simulink model "sedemo_absbrake_can"  (Simulink 7.5)
settings: Solver=ode45  SolverMode=SingleTasking  StartTime=0.0  StopTime=17  MaxStep=inf  RelTol=2e-2  AbsTol=1e-4
PreLoadFcn:
  | sedemo_absdata;
  | BUSCapacity = 50000;
StopFcn:
  | if exist ('logsout')
  | tagName = 'Net';
  | sedemo_absbrakeplots_delay;
  | clear figExt tagName;
  | end
values from neighbouring files (symbols this model uses):
  ctrl = 1    [sedemo_absdata.m]
  g = 32.18    [sedemo_absdata.m]
  I = 5    [sedemo_absdata.m]
  Kf = 1    [sedemo_absdata.m]
  m = 50    [sedemo_absdata.m]
  mu = [0 .4 .8 .97 1.0 .98 .96 .94 .92 .9 .88 .855 .83 .81 .79 .77 .75 .73 .72 .71 .7]    [sedemo_absdata.m]
  PBmax = 1500    [sedemo_absdata.m]
  Rr = 15/12    (= 1.25)    [sedemo_absdata.m]
  slip = (0:.05:1.0)    [sedemo_absdata.m]
  TB = 0.01    [sedemo_absdata.m]
  v0 = 88    [sedemo_absdata.m]
undefined symbols (not defined in the file or in its folder): des_subsystemblock, des_subsysteminport, des_subsystemoutport, des_subsystemsupportblock
libraries: simeventsrouting1 x30, simeventstranslate1 x25, simeventssink1 x21, simeventsserver1 x19, simeventsattributes2 x15, simeventsgates1 x10, simeventsqueue1 x6, simulink x5, simeventsgenerators1 x5, simeventssignalmanage1 x5, simeventstiming1 x3, simeventsinfo x1
(part 2 of 4)

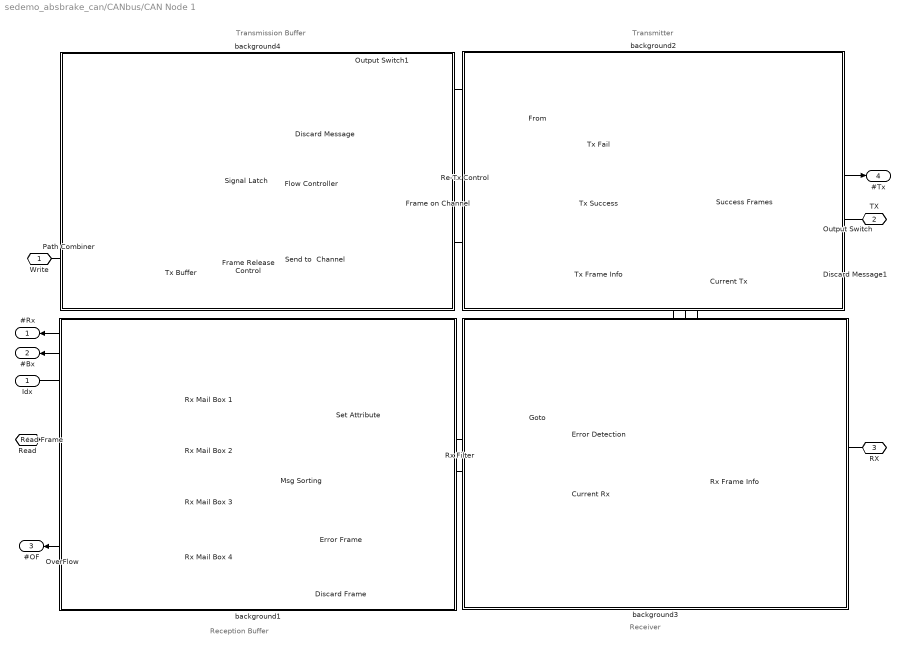
== system sedemo_absbrake_can/CANbus/CAN Node 1 ==
  note: Receiver
  note: Transmitter
  note: Transmission Buffer
  note: Reception Buffer
  Idx : Inport  OutDataType=sfix(16)  OutScaling=2^0
  Current Rx : simeventsserver1/Single Server  Priority=1  SystemSampleTime=-1  ServiceTimeFrom=Dialog  ServiceTime=0  AttributeName=ServiceTime  PriorityServiceCompletion=2400  PermitPreemption=off  SortingAttributeName=ID  SortingDirection=Ascending  WriteToAttribute=off  ResidualAttributeName=ResidualServiceTime  CreateAttribute=on  EnableTOPort=off  StatNumberDeparted=Off  StatNumberInBlock=Off  StatNumberPreempted=Off  StatPendingEntity=Off  StatAverageWait=Off  StatUtilization=Off  StatNumberTimedout=Off
  Current Tx : simeventsserver1/Single Server  Priority=1  SystemSampleTime=-1  ServiceTimeFrom=Dialog  ServiceTime=0  AttributeName=ServiceTime  PriorityServiceCompletion=2400  PermitPreemption=off  SortingAttributeName=ID  SortingDirection=Ascending  WriteToAttribute=off  ResidualAttributeName=ResidualServiceTime  CreateAttribute=on  EnableTOPort=off  StatNumberDeparted=Off  StatNumberInBlock=Off  StatNumberPreempted=Off  StatPendingEntity=Off  StatAverageWait=Off  StatUtilization=Off  StatNumberTimedout=Off
  Discard Message1 : simeventssink1/Entity Sink  Priority=1  SystemSampleTime=-1  AvailableForArrivals=on  StatNumberArrived=Off
  Discard Frame : simeventssink1/Entity Sink  Priority=1  SystemSampleTime=-1  AvailableForArrivals=on  StatNumberArrived=Off
  Discard Message : simeventssink1/Entity Sink  Priority=1  SystemSampleTime=-1  AvailableForArrivals=on  StatNumberArrived=Off
  Error Detection : Subsystem  LoadFcn=des_subsystemblock(gcb, 'load');  InitFcn=des_subsystemblock(gcb, 'init');  StartFcn=des_subsystemblock(gcb, 'start');  StopFcn=des_subsystemblock(gcb, 'stop');
      settings: CopyFcn=des_subsystemblock(gcb, 'copy');  DeleteFcn=des_subsystemblock(gcb, 'delete');  UndoDeleteFcn=des_subsystemblock(gcb, 'undodelete');  ModelCloseFcn=des_subsystemblock(gcb, 'modelclose');  PreSaveFcn=des_subsystemblock(gcb, 'presave');  NameChangeFcn=des_subsystemblock(gcb, 'namechange');  ParentCloseFcn=des_subsystemblock(gcb, 'parentclose');  ErrorFcn=des_subsystemerror
  Error Frame : simeventssink1/Entity Sink  Priority=1  SystemSampleTime=-1  AvailableForArrivals=on  StatNumberArrived=Off
  Flow Controller : Subsystem  LoadFcn=des_subsystemblock(gcb, 'load');  InitFcn=des_subsystemblock(gcb, 'init');  StartFcn=des_subsystemblock(gcb, 'start');  StopFcn=des_subsystemblock(gcb, 'stop');
      settings: CopyFcn=des_subsystemblock(gcb, 'copy');  DeleteFcn=des_subsystemblock(gcb, 'delete');  UndoDeleteFcn=des_subsystemblock(gcb, 'undodelete');  ModelCloseFcn=des_subsystemblock(gcb, 'modelclose');  PreSaveFcn=des_subsystemblock(gcb, 'presave');  NameChangeFcn=des_subsystemblock(gcb, 'namechange');  ParentCloseFcn=des_subsystemblock(gcb, 'parentclose');  ErrorFcn=des_subsystemerror
  Frame Release Control : simeventsgates1/Enabled Gate  Priority=1  SystemSampleTime=-1  SpecifyEventPriority=on  PriorityGateEnableOpenClose=2300  StatNumberDeparted=Off
  Frame on Channel : simeventsqueue1/FIFO Queue  Priority=1  SystemSampleTime=-1  Capacity=2  EnableTOPort=off  StatNumberDeparted=Off  StatNumberInBlock=On  StatPendingEntity=Off  StatAverageWait=Off  StatAverageQueueLength=Off  StatNumberTimedout=Off
  Msg Sorting : simeventsrouting1/Output Switch  Priority=1  SystemSampleTime=-1  NumberOutputPorts=4  SwitchingCriterion=Round robin  InitialSeed=34567  AttributeName=Attribute1  InitialConditionsOpt=off  InitialConditions=1  EntityBufferOpt=off  SpecifyEventPriority=off  PriorityOutputSwitchSelectPort=4100  TimeoutPortOpt=off  StatNumberDeparted=On  StatNumberTimedOut=Off  StatPendingEntity=Off  StatLastDeparturePort=On  EvaluatedNumPorts=4
  Output Switch : simeventsrouting1/Output Switch  Priority=1  SystemSampleTime=-1  NumberOutputPorts=2  SwitchingCriterion=First port that is not blocked  InitialSeed=34567  AttributeName=Attribute1  InitialConditionsOpt=off  InitialConditions=1  EntityBufferOpt=off  SpecifyEventPriority=off  PriorityOutputSwitchSelectPort=4100  TimeoutPortOpt=off  StatNumberDeparted=Off  StatNumberTimedOut=Off  StatPendingEntity=Off  StatLastDeparturePort=Off  EvaluatedNumPorts=2
  Output Switch1 : simeventsrouting1/Output Switch  Priority=1  SystemSampleTime=-1  NumberOutputPorts=2  SwitchingCriterion=First port that is not blocked  InitialSeed=34567  AttributeName=Attribute1  InitialConditionsOpt=off  InitialConditions=1  EntityBufferOpt=off  SpecifyEventPriority=off  PriorityOutputSwitchSelectPort=4100  TimeoutPortOpt=off  StatNumberDeparted=Off  StatNumberTimedOut=Off  StatPendingEntity=Off  StatLastDeparturePort=Off  EvaluatedNumPorts=2
  OverFlow : simeventsrouting1/Path Combiner  Priority=1  SystemSampleTime=-1  NumberInputPorts=4  InputPortPrecedence=IN1 port  InitialSeed=45675  SpecifyEventPriority=off  PriorityPathCombinerPortPrecedenceSelection=4100  StatNumberDeparted=On  StatLastArrivalPort=Off  EvaluatedNumPorts=4
  Path Combiner : simeventsrouting1/Path Combiner  Priority=1  SystemSampleTime=-1  NumberInputPorts=2  InputPortPrecedence=IN1 port  InitialSeed=45675  SpecifyEventPriority=off  PriorityPathCombinerPortPrecedenceSelection=4100  StatNumberDeparted=Off  StatLastArrivalPort=Off  EvaluatedNumPorts=2
  Re-Tx Control : simeventsrouting1/Output Switch  Priority=1  SystemSampleTime=-1  NumberOutputPorts=2  SwitchingCriterion=First port that is not blocked  InitialSeed=34567  AttributeName=Attribute1  InitialConditionsOpt=off  InitialConditions=1  EntityBufferOpt=off  SpecifyEventPriority=off  PriorityOutputSwitchSelectPort=4100  TimeoutPortOpt=off  StatNumberDeparted=Off  StatNumberTimedOut=Off  StatPendingEntity=Off  StatLastDeparturePort=Off  EvaluatedNumPorts=2
  Read Frame : simeventsrouting1/Input Switch  Priority=1  SystemSampleTime=-1  NumberInputPorts=4  SwitchingCriterion=From signal port p  InitialSeed=23453  SpecifyEventPriority=off  PriorityInputSwitchSelectPort=4000  StatNumberDeparted=Off  StatLastArrivalPort=Off  EvaluatedNumPorts=4
  Rx Filter : simeventsrouting1/Output Switch  Priority=1  SystemSampleTime=-1  NumberOutputPorts=3  SwitchingCriterion=From signal port p  InitialSeed=34567  AttributeName=Attribute1  InitialConditionsOpt=off  InitialConditions=1  EntityBufferOpt=off  SpecifyEventPriority=off  PriorityOutputSwitchSelectPort=4100  TimeoutPortOpt=off  StatNumberDeparted=On  StatNumberTimedOut=Off  StatPendingEntity=Off  StatLastDeparturePort=Off  EvaluatedNumPorts=3
  Rx Frame Info : simeventsattributes2/Get Attribute  Priority=1  DialogController=des_ddg_create  DialogControllerArgs=DataTag128  SystemSampleTime=-1  AttributeName=ID|RndLoss|RTR|Data  AttributeMissing=Error|Error|Error|Error  AttributeDefaultValue=1|1|1|1  AttributeSendTiming=After entity departure|After entity departure|After entity departure|After entity departure  AttributeTreatAsVector=1|1|1|1  StatNumberDeparted=Off  EvaluatedDefaultAttributeValue={[];[];[];[]}
  Rx Mail Box {1..4} (4 alike) : simeventsserver1/Single Server  Priority=1  SystemSampleTime=-1  ServiceTimeFrom=Dialog  ServiceTime=0  AttributeName=ServiceTime  PriorityServiceCompletion=2400  PermitPreemption=on  SortingAttributeName=time  SortingDirection=Descending  WriteToAttribute=off  ResidualAttributeName=ResidualServiceTime  CreateAttribute=on  EnableTOPort=off  StatNumberDeparted=Off  StatNumberInBlock=Off  StatNumberPreempted=Off  StatPendingEntity=Off  StatAverageWait=Off  StatUtilization=Off  StatNumberTimedout=Off
  Send to  Channel : simeventsrouting1/Replicate  Priority=1  SystemSampleTime=-1  NumberOutputPorts=2  ReplicateEntityWhen=All entity output ports are not blocked  OutputPortPrecedence=OUT1 port  InitialSeed=56789  ActionUponBlocking=Discard entity  StatNumberArrived=Off  StatNumberDeparted=Off  EvaluatedNumPorts=2
  Set Attribute : simeventsattributes2/Set Attribute  Priority=1  DialogController=des_ddg_create  DialogControllerArgs=DataTag135  SystemSampleTime=-1  AttributeFrom=Signal port  AttributeName=time  AttributeTreatAsVector=1  AttributeValue=1  AttributeCreate=on  StatNumberDeparted=Off  EvaluatedAttributeValue={[]}
  Signal Latch : simeventssignalmanage1/Signal Latch  Priority=1  SystemSampleTime=-1  InitialMemoryValue=1  WriteMemoryUpon=Sample time hit from port wts  MemoryWriteEdgeOption=Either  SpecifyWriteEventPriority=on  PriorityMemoryWrite=2200  ReadMemoryUpon=Write to memory event  MemoryReadEdgeOption=Falling  SpecifyReadEventPriority=on  PriorityMemoryRead=7000  ReportMemoryState=off  ReportMemoryUponWrite=off  ReportMemoryUponRead=on
  Success Frames : simeventssink1/Entity Sink  Priority=1  SystemSampleTime=-1  AvailableForArrivals=on  StatNumberArrived=On
  Tx Buffer : simeventsqueue1/Priority Queue  Priority=1  SystemSampleTime=-1  Capacity=15  SortingAttributeName=ID  SortingDirection=Ascending  EnableTOPort=off  StatNumberDeparted=Off  StatNumberInBlock=Off  StatPendingEntity=Off  StatAverageWait=Off  StatAverageQueueLength=Off  StatNumberTimedout=Off
  Tx Fail : simeventsgates1/Release Gate  Priority=1  SystemSampleTime=-1  OpenGateUpon=Change in signal from port vc  SignalEdgeOption=Falling  SpecifyEventPriority=on  PriorityGateRelease=2000  StatNumberDeparted=Off
  Tx Frame Info : simeventsattributes2/Get Attribute  Priority=1  DialogController=des_ddg_create  DialogControllerArgs=DataTag141  SystemSampleTime=-1  AttributeName=ID|RTR|Data  AttributeMissing=Error|Error|Error  AttributeDefaultValue=1|1|1  AttributeSendTiming=After entity departure|After entity departure|After entity departure  AttributeTreatAsVector=1|1|1  StatNumberDeparted=Off  EvaluatedDefaultAttributeValue={[];[];[]}
  Tx Success : simeventsgates1/Release Gate  Priority=1  SystemSampleTime=-1  OpenGateUpon=Change in signal from port vc  SignalEdgeOption=Rising  SpecifyEventPriority=on  PriorityGateRelease=2000  StatNumberDeparted=Off
  background1 : Subsystem
      mask Display: disp('')
  background2 : Subsystem
      mask Display: disp('')
  background3 : Subsystem
      mask Display: disp('')
  background4 : Subsystem
      mask Display: disp('')
  Write : PMIOPort  Port=1  Side=Right
  TX : PMIOPort  Port=2  Side=Left
  RX : PMIOPort  Port=3  Side=Left
  Read : PMIOPort  Port=4  Side=Right
  #Rx : Outport  OutDataType=sfix(16)  OutScaling=2^0
  #Bx : Outport  Port=2  OutDataType=sfix(16)  OutScaling=2^0
  #OF : Outport  Port=3  OutDataType=sfix(16)  OutScaling=2^0
  #Tx : Outport  Port=4  OutDataType=sfix(16)  OutScaling=2^0
  wires:
  [Ack] -> Tx Success/1, Tx Fail/1
  Error Detection/2(ACK) -> [Ack]
  Error Detection/1(Idx) -> Rx Filter/1
  Rx Frame Info/4 -> Error Detection/4(Rx_Data)
  Rx Frame Info/3 -> Error Detection/3(Rx_RTR)
  Tx Frame Info/1 -> Error Detection/5(Tx_ID)
  Tx Frame Info/2 -> Error Detection/6(Tx_RTR)
  Tx Frame Info/3 -> Error Detection/7(Tx_Data)
  Rx Frame Info/2 -> Error Detection/2(Loss)
  Rx Frame Info/1 -> Error Detection/1(Rx_ID)
  Rx Filter/1 -> Set Attribute/1
  Frame on Channel/1 -> Flow Controller/1(busy)
  Idx/1 -> Read Frame/1
  Msg Sorting/2 -> #Bx/1
  OverFlow/1 -> #OF/1
  Msg Sorting/1 -> #Rx/1
  Success Frames/1 -> #Tx/1
  Flow Controller/1(en) -> Signal Latch/1, Signal Latch/2
  Signal Latch/1 -> Frame Release Control/1
  connections:
  Tx Frame Info/RConn1 -- Current Tx/LConn1
  Current Tx/RConn1 -- Output Switch/LConn1
  Send to  Channel/RConn1 -- Frame on Channel/LConn1
  Send to  Channel/RConn2 -- Tx Frame Info/LConn1
  RX/RConn1 -- Rx Frame Info/LConn1
  Rx Mail Box 4/RConn1 -- Read Frame/LConn4
  Rx Mail Box 3/RConn1 -- Read Frame/LConn3
  Rx Mail Box 2/RConn1 -- Read Frame/LConn2
  Rx Mail Box 1/RConn1 -- Read Frame/LConn1
  Rx Mail Box 1/RConn2 -- OverFlow/LConn1
  Rx Mail Box 2/RConn2 -- OverFlow/LConn2
  Rx Mail Box 3/RConn2 -- OverFlow/LConn3
  Rx Mail Box 4/RConn2 -- OverFlow/LConn4
  Rx Frame Info/RConn1 -- Current Rx/LConn1
  Output Switch1/RConn1 -- Path Combiner/LConn1
  Tx Fail/RConn1 -- Output Switch1/LConn1
  Output Switch/RConn1 -- TX/RConn1
  Set Attribute/RConn1 -- Msg Sorting/LConn1
  Rx Filter/RConn1 -- Set Attribute/LConn1
  Rx Filter/RConn3 -- Discard Frame/LConn1
  Tx Success/RConn1 -- Success Frames/LConn1
  Write/RConn1 -- Path Combiner/LConn2
  Path Combiner/RConn1 -- Tx Buffer/LConn1
  Frame Release Control/RConn1 -- Send to  Channel/LConn1
  Tx Buffer/RConn1 -- Frame Release Control/LConn1
  Re-Tx Control/RConn1 -- Tx Fail/LConn1
  Re-Tx Control/RConn2 -- Tx Success/LConn1
  Frame on Channel/RConn1 -- Re-Tx Control/LConn1
  Current Rx/RConn1 -- Rx Filter/LConn1
  Rx Filter/RConn2 -- Error Frame/LConn1
  Msg Sorting/RConn1 -- Rx Mail Box 1/LConn1
  Msg Sorting/RConn2 -- Rx Mail Box 2/LConn1
  Msg Sorting/RConn3 -- Rx Mail Box 3/LConn1
  Msg Sorting/RConn4 -- Rx Mail Box 4/LConn1
  Read Frame/RConn1 -- Read/RConn1
  Output Switch/RConn2 -- Discard Message1/LConn1
  Discard Message/LConn1 -- Output Switch1/RConn2

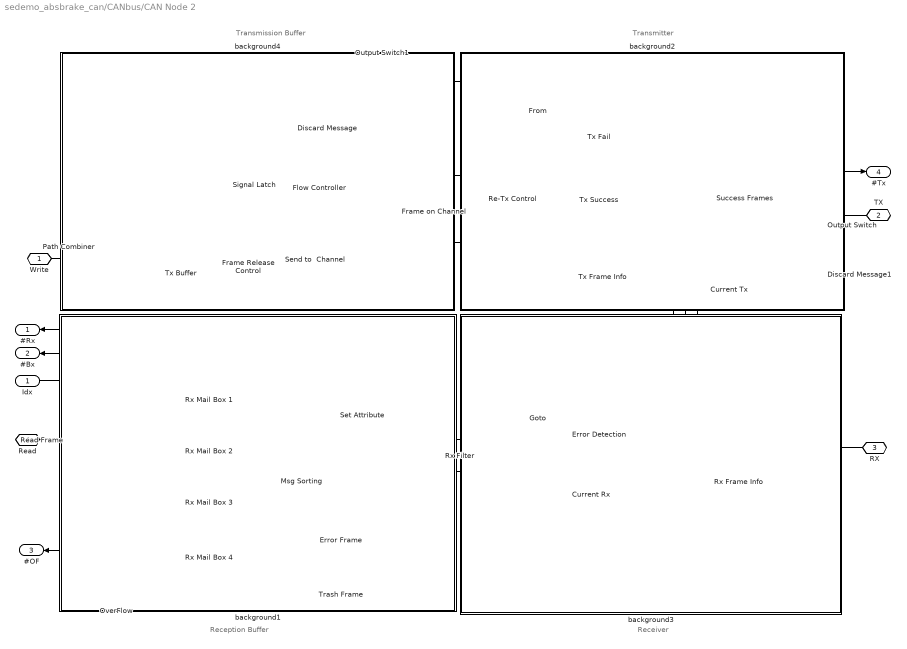
== system sedemo_absbrake_can/CANbus/CAN Node 2 ==
  note: Receiver
  note: Transmitter
  note: Transmission Buffer
  note: Reception Buffer
  Idx : Inport  OutDataType=sfix(16)  OutScaling=2^0
  Current Rx : simeventsserver1/Single Server  Priority=1  SystemSampleTime=-1  ServiceTimeFrom=Dialog  ServiceTime=0  AttributeName=ServiceTime  PriorityServiceCompletion=2400  PermitPreemption=off  SortingAttributeName=ID  SortingDirection=Ascending  WriteToAttribute=off  ResidualAttributeName=ResidualServiceTime  CreateAttribute=on  EnableTOPort=off  StatNumberDeparted=Off  StatNumberInBlock=Off  StatNumberPreempted=Off  StatPendingEntity=Off  StatAverageWait=Off  StatUtilization=Off  StatNumberTimedout=Off
  Current Tx : simeventsserver1/Single Server  Priority=1  SystemSampleTime=-1  ServiceTimeFrom=Dialog  ServiceTime=0  AttributeName=ServiceTime  PriorityServiceCompletion=2400  PermitPreemption=off  SortingAttributeName=ID  SortingDirection=Ascending  WriteToAttribute=off  ResidualAttributeName=ResidualServiceTime  CreateAttribute=on  EnableTOPort=off  StatNumberDeparted=Off  StatNumberInBlock=Off  StatNumberPreempted=Off  StatPendingEntity=Off  StatAverageWait=Off  StatUtilization=Off  StatNumberTimedout=Off
  Discard Message : simeventssink1/Entity Sink  Priority=1  SystemSampleTime=-1  AvailableForArrivals=on  StatNumberArrived=Off
  Discard Message1 : simeventssink1/Entity Sink  Priority=1  SystemSampleTime=-1  AvailableForArrivals=on  StatNumberArrived=Off
  Error Detection : Subsystem  LoadFcn=des_subsystemblock(gcb, 'load');  InitFcn=des_subsystemblock(gcb, 'init');  StartFcn=des_subsystemblock(gcb, 'start');  StopFcn=des_subsystemblock(gcb, 'stop');
      settings: CopyFcn=des_subsystemblock(gcb, 'copy');  DeleteFcn=des_subsystemblock(gcb, 'delete');  UndoDeleteFcn=des_subsystemblock(gcb, 'undodelete');  ModelCloseFcn=des_subsystemblock(gcb, 'modelclose');  PreSaveFcn=des_subsystemblock(gcb, 'presave');  NameChangeFcn=des_subsystemblock(gcb, 'namechange');  ParentCloseFcn=des_subsystemblock(gcb, 'parentclose');  ErrorFcn=des_subsystemerror
  Error Frame : simeventssink1/Entity Sink  Priority=1  SystemSampleTime=-1  AvailableForArrivals=on  StatNumberArrived=Off
  Flow Controller : Subsystem  LoadFcn=des_subsystemblock(gcb, 'load');  InitFcn=des_subsystemblock(gcb, 'init');  StartFcn=des_subsystemblock(gcb, 'start');  StopFcn=des_subsystemblock(gcb, 'stop');
      settings: CopyFcn=des_subsystemblock(gcb, 'copy');  DeleteFcn=des_subsystemblock(gcb, 'delete');  UndoDeleteFcn=des_subsystemblock(gcb, 'undodelete');  ModelCloseFcn=des_subsystemblock(gcb, 'modelclose');  PreSaveFcn=des_subsystemblock(gcb, 'presave');  NameChangeFcn=des_subsystemblock(gcb, 'namechange');  ParentCloseFcn=des_subsystemblock(gcb, 'parentclose');  ErrorFcn=des_subsystemerror
  Frame Release Control : simeventsgates1/Enabled Gate  Priority=1  SystemSampleTime=-1  SpecifyEventPriority=on  PriorityGateEnableOpenClose=2300  StatNumberDeparted=Off
  Frame on Channel : simeventsqueue1/FIFO Queue  Priority=1  SystemSampleTime=-1  Capacity=2  EnableTOPort=off  StatNumberDeparted=Off  StatNumberInBlock=On  StatPendingEntity=Off  StatAverageWait=Off  StatAverageQueueLength=Off  StatNumberTimedout=Off
  Msg Sorting : simeventsrouting1/Output Switch  Priority=1  SystemSampleTime=-1  NumberOutputPorts=4  SwitchingCriterion=Round robin  InitialSeed=34567  AttributeName=Attribute1  InitialConditionsOpt=off  InitialConditions=1  EntityBufferOpt=off  SpecifyEventPriority=off  PriorityOutputSwitchSelectPort=4100  TimeoutPortOpt=off  StatNumberDeparted=On  StatNumberTimedOut=Off  StatPendingEntity=Off  StatLastDeparturePort=On  EvaluatedNumPorts=4
  Output Switch : simeventsrouting1/Output Switch  Priority=1  SystemSampleTime=-1  NumberOutputPorts=2  SwitchingCriterion=First port that is not blocked  InitialSeed=34567  AttributeName=Attribute1  InitialConditionsOpt=off  InitialConditions=1  EntityBufferOpt=off  SpecifyEventPriority=off  PriorityOutputSwitchSelectPort=4100  TimeoutPortOpt=off  StatNumberDeparted=Off  StatNumberTimedOut=Off  StatPendingEntity=Off  StatLastDeparturePort=Off  EvaluatedNumPorts=2
  Output Switch1 : simeventsrouting1/Output Switch  Priority=1  SystemSampleTime=-1  NumberOutputPorts=2  SwitchingCriterion=First port that is not blocked  InitialSeed=34567  AttributeName=Attribute1  InitialConditionsOpt=off  InitialConditions=1  EntityBufferOpt=off  SpecifyEventPriority=off  PriorityOutputSwitchSelectPort=4100  TimeoutPortOpt=off  StatNumberDeparted=Off  StatNumberTimedOut=Off  StatPendingEntity=Off  StatLastDeparturePort=Off  EvaluatedNumPorts=2
  OverFlow : simeventsrouting1/Path Combiner  Priority=1  SystemSampleTime=-1  NumberInputPorts=4  InputPortPrecedence=IN1 port  InitialSeed=45675  SpecifyEventPriority=off  PriorityPathCombinerPortPrecedenceSelection=4100  StatNumberDeparted=On  StatLastArrivalPort=Off  EvaluatedNumPorts=4
  Path Combiner : simeventsrouting1/Path Combiner  Priority=1  SystemSampleTime=-1  NumberInputPorts=2  InputPortPrecedence=IN1 port  InitialSeed=45675  SpecifyEventPriority=off  PriorityPathCombinerPortPrecedenceSelection=4100  StatNumberDeparted=Off  StatLastArrivalPort=Off  EvaluatedNumPorts=2
  Re-Tx Control : simeventsrouting1/Output Switch  Priority=1  SystemSampleTime=-1  NumberOutputPorts=2  SwitchingCriterion=First port that is not blocked  InitialSeed=34567  AttributeName=Attribute1  InitialConditionsOpt=off  InitialConditions=1  EntityBufferOpt=off  SpecifyEventPriority=off  PriorityOutputSwitchSelectPort=4100  TimeoutPortOpt=off  StatNumberDeparted=Off  StatNumberTimedOut=Off  StatPendingEntity=Off  StatLastDeparturePort=Off  EvaluatedNumPorts=2
  Read Frame : simeventsrouting1/Input Switch  Priority=1  SystemSampleTime=-1  NumberInputPorts=4  SwitchingCriterion=From signal port p  InitialSeed=23453  SpecifyEventPriority=off  PriorityInputSwitchSelectPort=4000  StatNumberDeparted=Off  StatLastArrivalPort=Off  EvaluatedNumPorts=4
  Rx Filter : simeventsrouting1/Output Switch  Priority=1  SystemSampleTime=-1  NumberOutputPorts=3  SwitchingCriterion=From signal port p  InitialSeed=34567  AttributeName=Attribute1  InitialConditionsOpt=off  InitialConditions=1  EntityBufferOpt=off  SpecifyEventPriority=off  PriorityOutputSwitchSelectPort=4100  TimeoutPortOpt=off  StatNumberDeparted=On  StatNumberTimedOut=Off  StatPendingEntity=Off  StatLastDeparturePort=Off  EvaluatedNumPorts=3
  Rx Frame Info : simeventsattributes2/Get Attribute  Priority=1  DialogController=des_ddg_create  DialogControllerArgs=DataTag186  SystemSampleTime=-1  AttributeName=ID|RndLoss|RTR|Data  AttributeMissing=Error|Error|Error|Error  AttributeDefaultValue=1|1|1|1  AttributeSendTiming=After entity departure|After entity departure|After entity departure|After entity departure  AttributeTreatAsVector=1|1|1|1  StatNumberDeparted=Off  EvaluatedDefaultAttributeValue={[];[];[];[]}
  Rx Mail Box {1..4} (4 alike) : simeventsserver1/Single Server  Priority=1  SystemSampleTime=-1  ServiceTimeFrom=Dialog  ServiceTime=0  AttributeName=ServiceTime  PriorityServiceCompletion=2400  PermitPreemption=on  SortingAttributeName=time  SortingDirection=Descending  WriteToAttribute=off  ResidualAttributeName=ResidualServiceTime  CreateAttribute=on  EnableTOPort=off  StatNumberDeparted=Off  StatNumberInBlock=Off  StatNumberPreempted=Off  StatPendingEntity=Off  StatAverageWait=Off  StatUtilization=Off  StatNumberTimedout=Off
  Send to  Channel : simeventsrouting1/Replicate  Priority=1  SystemSampleTime=-1  NumberOutputPorts=2  ReplicateEntityWhen=All entity output ports are not blocked  OutputPortPrecedence=OUT1 port  InitialSeed=56789  ActionUponBlocking=Discard entity  StatNumberArrived=Off  StatNumberDeparted=Off  EvaluatedNumPorts=2
  Set Attribute : simeventsattributes2/Set Attribute  Priority=1  DialogController=des_ddg_create  DialogControllerArgs=DataTag193  SystemSampleTime=-1  AttributeFrom=Signal port  AttributeName=time  AttributeTreatAsVector=1  AttributeValue=1  AttributeCreate=on  StatNumberDeparted=Off  EvaluatedAttributeValue={[]}
  Signal Latch : simeventssignalmanage1/Signal Latch  Priority=1  SystemSampleTime=-1  InitialMemoryValue=1  WriteMemoryUpon=Sample time hit from port wts  MemoryWriteEdgeOption=Either  SpecifyWriteEventPriority=on  PriorityMemoryWrite=2200  ReadMemoryUpon=Write to memory event  MemoryReadEdgeOption=Falling  SpecifyReadEventPriority=on  PriorityMemoryRead=7000  ReportMemoryState=off  ReportMemoryUponWrite=off  ReportMemoryUponRead=on
  Success Frames : simeventssink1/Entity Sink  Priority=1  SystemSampleTime=-1  AvailableForArrivals=on  StatNumberArrived=On
  Trash Frame : simeventssink1/Entity Sink  Priority=1  SystemSampleTime=-1  AvailableForArrivals=on  StatNumberArrived=Off
  Tx Buffer : simeventsqueue1/Priority Queue  Priority=1  SystemSampleTime=-1  Capacity=15  SortingAttributeName=ID  SortingDirection=Ascending  EnableTOPort=off  StatNumberDeparted=Off  StatNumberInBlock=Off  StatPendingEntity=Off  StatAverageWait=Off  StatAverageQueueLength=Off  StatNumberTimedout=Off
  Tx Fail : simeventsgates1/Release Gate  Priority=1  SystemSampleTime=-1  OpenGateUpon=Change in signal from port vc  SignalEdgeOption=Falling  SpecifyEventPriority=on  PriorityGateRelease=2000  StatNumberDeparted=Off
  Tx Frame Info : simeventsattributes2/Get Attribute  Priority=1  DialogController=des_ddg_create  DialogControllerArgs=DataTag200  SystemSampleTime=-1  AttributeName=ID|RTR|Data  AttributeMissing=Error|Error|Error  AttributeDefaultValue=1|1|1  AttributeSendTiming=After entity departure|After entity departure|After entity departure  AttributeTreatAsVector=1|1|1  StatNumberDeparted=Off  EvaluatedDefaultAttributeValue={[];[];[]}
  Tx Success : simeventsgates1/Release Gate  Priority=1  SystemSampleTime=-1  OpenGateUpon=Change in signal from port vc  SignalEdgeOption=Rising  SpecifyEventPriority=on  PriorityGateRelease=2000  StatNumberDeparted=Off
  background1 : Subsystem
      mask Display: disp('')
  background2 : Subsystem
      mask Display: disp('')
  background3 : Subsystem
      mask Display: disp('')
  background4 : Subsystem
      mask Display: disp('')
  Write : PMIOPort  Port=1  Side=Right
  TX : PMIOPort  Port=2  Side=Left
  RX : PMIOPort  Port=3  Side=Left
  Read : PMIOPort  Port=4  Side=Right
  #Rx : Outport  OutDataType=sfix(16)  OutScaling=2^0
  #Bx : Outport  Port=2  OutDataType=sfix(16)  OutScaling=2^0
  #OF : Outport  Port=3  OutDataType=sfix(16)  OutScaling=2^0
  #Tx : Outport  Port=4  OutDataType=sfix(16)  OutScaling=2^0
  wires:
  [Ack] -> Tx Success/1, Tx Fail/1
  Error Detection/2(ACK) -> [Ack]
  Error Detection/1(Idx) -> Rx Filter/1
  Rx Frame Info/4 -> Error Detection/4(Rx_Data)
  Rx Frame Info/3 -> Error Detection/3(Rx_RTR)
  Tx Frame Info/1 -> Error Detection/5(Tx_ID)
  Tx Frame Info/2 -> Error Detection/6(Tx_RTR)
  Tx Frame Info/3 -> Error Detection/7(Tx_Data)
  Rx Frame Info/2 -> Error Detection/2(Loss)
  Rx Frame Info/1 -> Error Detection/1(Rx_ID)
  Rx Filter/1 -> Set Attribute/1
  Frame on Channel/1 -> Flow Controller/1(busy)
  Signal Latch/1 -> Frame Release Control/1
  Idx/1 -> Read Frame/1
  Msg Sorting/2 -> #Bx/1
  OverFlow/1 -> #OF/1
  Msg Sorting/1 -> #Rx/1
  Success Frames/1 -> #Tx/1
  Flow Controller/1(en) -> Signal Latch/1, Signal Latch/2
  connections:
  Tx Frame Info/RConn1 -- Current Tx/LConn1
  Current Tx/RConn1 -- Output Switch/LConn1
  Send to  Channel/RConn1 -- Frame on Channel/LConn1
  Send to  Channel/RConn2 -- Tx Frame Info/LConn1
  RX/RConn1 -- Rx Frame Info/LConn1
  Rx Mail Box 4/RConn1 -- Read Frame/LConn4
  Rx Mail Box 3/RConn1 -- Read Frame/LConn3
  Rx Mail Box 2/RConn1 -- Read Frame/LConn2
  Rx Mail Box 1/RConn1 -- Read Frame/LConn1
  Rx Mail Box 1/RConn2 -- OverFlow/LConn1
  Rx Mail Box 2/RConn2 -- OverFlow/LConn2
  Rx Mail Box 3/RConn2 -- OverFlow/LConn3
  Rx Mail Box 4/RConn2 -- OverFlow/LConn4
  Rx Frame Info/RConn1 -- Current Rx/LConn1
  Output Switch1/RConn1 -- Path Combiner/LConn1
  Tx Fail/RConn1 -- Output Switch1/LConn1
  Output Switch/RConn1 -- TX/RConn1
  Set Attribute/RConn1 -- Msg Sorting/LConn1
  Rx Filter/RConn1 -- Set Attribute/LConn1
  Rx Filter/RConn3 -- Trash Frame/LConn1
  Tx Success/RConn1 -- Success Frames/LConn1
  Write/RConn1 -- Path Combiner/LConn2
  Path Combiner/RConn1 -- Tx Buffer/LConn1
  Frame Release Control/RConn1 -- Send to  Channel/LConn1
  Tx Buffer/RConn1 -- Frame Release Control/LConn1
  Re-Tx Control/RConn1 -- Tx Fail/LConn1
  Re-Tx Control/RConn2 -- Tx Success/LConn1
  Frame on Channel/RConn1 -- Re-Tx Control/LConn1
  Current Rx/RConn1 -- Rx Filter/LConn1
  Rx Filter/RConn2 -- Error Frame/LConn1
  Msg Sorting/RConn1 -- Rx Mail Box 1/LConn1
  Msg Sorting/RConn2 -- Rx Mail Box 2/LConn1
  Msg Sorting/RConn3 -- Rx Mail Box 3/LConn1
  Msg Sorting/RConn4 -- Rx Mail Box 4/LConn1
  Read Frame/RConn1 -- Read/RConn1
  Discard Message/LConn1 -- Output Switch1/RConn2
  Output Switch/RConn2 -- Discard Message1/LConn1

== system sedemo_absbrake_can/CANbus/Msg Definition ==
  RTR : Inport  OutDataType=sfix(16)  OutScaling=2^0
  Data : Inport  Port=2  OutDataType=sfix(16)  OutScaling=2^0
  CommDelay : Constant  Value=(49+8*MsgSize)/BUSCapacity  OutDataType=sfix(16)  OutScaling=2^0
  ID : Constant  Value=MsgID  OutDataType=sfix(16)  OutScaling=2^0
  Set Attribute : simeventsattributes2/Set Attribute  Priority=1  DialogController=des_ddg_create  DialogControllerArgs=DataTag208  SystemSampleTime=-1  AttributeFrom=Signal port|Signal port|Signal port|Signal port|Signal port  AttributeName=ID|RTR|Size|Data|CommDelay  AttributeTreatAsVector=1|1|1|1|1  AttributeValue=1|1|1|1|1  AttributeCreate=on  StatNumberDeparted=Off  EvaluatedAttributeValue={[];[];[];[];[]}
  Size : Constant  Value=MsgSize  OutDataType=sfix(16)  OutScaling=2^0
  MsgOUT : PMIOPort  Port=1  Side=Right
  MsgIN : PMIOPort  Port=2  Side=Left
  wires:
  Data/1 -> Set Attribute/4
  RTR/1 -> Set Attribute/2
  Size/1 -> Set Attribute/3
  ID/1 -> Set Attribute/1
  CommDelay/1 -> Set Attribute/5
  connections:
  MsgIN/RConn1 -- Set Attribute/LConn1
  Set Attribute/RConn1 -- MsgOUT/RConn1

== system sedemo_absbrake_can/CANbus/Msg Definition1 ==
  RTR : Inport  OutDataType=sfix(16)  OutScaling=2^0
  Data : Inport  Port=2  OutDataType=sfix(16)  OutScaling=2^0
  CommDelay : Constant  Value=(49+8*MsgSize)/BUSCapacity  OutDataType=sfix(16)  OutScaling=2^0
  ID : Constant  Value=MsgID  OutDataType=sfix(16)  OutScaling=2^0
  Set Attribute : simeventsattributes2/Set Attribute  Priority=1  DialogController=des_ddg_create  DialogControllerArgs=DataTag210  SystemSampleTime=-1  AttributeFrom=Signal port|Signal port|Signal port|Signal port|Signal port  AttributeName=ID|RTR|Size|Data|CommDelay  AttributeTreatAsVector=1|1|1|1|1  AttributeValue=1|1|1|1|1  AttributeCreate=on  StatNumberDeparted=Off  EvaluatedAttributeValue={[];[];[];[];[]}
  Size : Constant  Value=MsgSize  OutDataType=sfix(16)  OutScaling=2^0
  MsgOUT : PMIOPort  Port=1  Side=Right
  MsgIN : PMIOPort  Port=2  Side=Left
  wires:
  Data/1 -> Set Attribute/4
  RTR/1 -> Set Attribute/2
  Size/1 -> Set Attribute/3
  ID/1 -> Set Attribute/1
  CommDelay/1 -> Set Attribute/5
  connections:
  MsgIN/RConn1 -- Set Attribute/LConn1
  Set Attribute/RConn1 -- MsgOUT/RConn1

== system sedemo_absbrake_can/CANbus/background1 ==

== system sedemo_absbrake_can/CANbus/background2 ==

== system sedemo_absbrake_can/CANbus/background8 ==

== system sedemo_absbrake_can/CANbus/Background Msg/Exponential  Interarrival 1 ==
  rate : Inport  OutDataType=sfix(16)  OutScaling=2^0
  Constant : Constant  OutDataType=sfix(16)  OutScaling=2^0
  Divide : Product  Inputs=*/  OutDataType=sfix(16)  OutScaling=2^-10
  Math Function : Math  Operator=log  OutDataType=sfix(16)  OutScaling=2^0  SaturateOnIntegerOverflow=on
  Product : Product  OutDataType=sfix(16)  OutScaling=2^0  RndMeth=Zero
  Subtract : Sum  Inputs=+-  OutDataType=sfix(16)  OutScaling=2^-10
  Unary Minus : simulink/Math Operations/Unary Minus  DoSatur=off
  Uniform Random Number : UniformRandomNumber  Minimum=0  Seed=seed  SampleTime=0
  Out1 : Outport  OutDataType=sfix(16)  OutScaling=2^0
  wires:
  Unary Minus/1 -> Out1/1
  Product/1 -> Unary Minus/1
  Math Function/1 -> Product/2
  Subtract/1 -> Math Function/1
  Uniform Random Number/1 -> Subtract/2
  Constant/1 -> Subtract/1, Divide/1
  rate/1 -> Divide/2
  Divide/1 -> Product/1

== system sedemo_absbrake_can/CANbus/Background Msg/Msg Definition1 ==
  RTR : Inport  OutDataType=sfix(16)  OutScaling=2^0
  Data : Inport  Port=2  OutDataType=sfix(16)  OutScaling=2^0
  CommDelay : Constant  Value=(49+8*MsgSize)/BUSCapacity  OutDataType=sfix(16)  OutScaling=2^0
  ID : Constant  Value=MsgID  OutDataType=sfix(16)  OutScaling=2^0
  Set Attribute : simeventsattributes2/Set Attribute  Priority=1  DialogController=des_ddg_create  DialogControllerArgs=DataTag1  SystemSampleTime=-1  AttributeFrom=Signal port|Signal port|Signal port|Signal port|Signal port  AttributeName=ID|RTR|Size|Data|CommDelay  AttributeTreatAsVector=1|1|1|1|1  AttributeValue=1|1|1|1|1  AttributeCreate=on  StatNumberDeparted=Off  EvaluatedAttributeValue={[];[];[];[];[]}
  Size : Constant  Value=MsgSize  OutDataType=sfix(16)  OutScaling=2^0
  MsgOUT : PMIOPort  Port=1  Side=Right
  MsgIN : PMIOPort  Port=2  Side=Left
  wires:
  ID/1 -> Set Attribute/1
  Size/1 -> Set Attribute/3
  RTR/1 -> Set Attribute/2
  Data/1 -> Set Attribute/4
  CommDelay/1 -> Set Attribute/5
  connections:
  Set Attribute/RConn1 -- MsgOUT/RConn1
  MsgIN/RConn1 -- Set Attribute/LConn1

== system sedemo_absbrake_can/CANbus/Background Msg/Msg Definition2 ==
  RTR : Inport  OutDataType=sfix(16)  OutScaling=2^0
  Data : Inport  Port=2  OutDataType=sfix(16)  OutScaling=2^0
  CommDelay : Constant  Value=(49+8*MsgSize)/BUSCapacity  OutDataType=sfix(16)  OutScaling=2^0
  ID : Constant  Value=MsgID  OutDataType=sfix(16)  OutScaling=2^0
  Set Attribute : simeventsattributes2/Set Attribute  Priority=1  DialogController=des_ddg_create  DialogControllerArgs=DataTag3  SystemSampleTime=-1  AttributeFrom=Signal port|Signal port|Signal port|Signal port|Signal port  AttributeName=ID|RTR|Size|Data|CommDelay  AttributeTreatAsVector=1|1|1|1|1  AttributeValue=1|1|1|1|1  AttributeCreate=on  StatNumberDeparted=Off  EvaluatedAttributeValue={[];[];[];[];[]}
  Size : Constant  Value=MsgSize  OutDataType=sfix(16)  OutScaling=2^0
  MsgOUT : PMIOPort  Port=1  Side=Right
  MsgIN : PMIOPort  Port=2  Side=Left
  wires:
  ID/1 -> Set Attribute/1
  Size/1 -> Set Attribute/3
  RTR/1 -> Set Attribute/2
  Data/1 -> Set Attribute/4
  CommDelay/1 -> Set Attribute/5
  connections:
  MsgIN/RConn1 -- Set Attribute/LConn1
  Set Attribute/RConn1 -- MsgOUT/RConn1

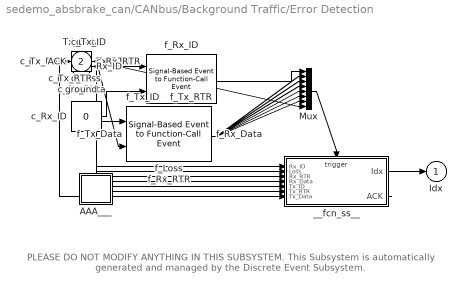
== system sedemo_absbrake_can/CANbus/Background Traffic/Error Detection ==
  note: PLEASE DO NOT MODIFY ANYTHING IN THIS SUBSYSTEM.
      | This Subsystem is automatically generated and
      | managed by the Discrete Event Subsystem.
  Rx_ID : Inport  DataType=double  OutDataType=sfix(16)  OutScaling=2^0  OutDataTypeStr=double
  Loss : Inport  Port=2  DataType=double  OutDataType=sfix(16)  OutScaling=2^0  OutDataTypeStr=double
  Rx_RTR : Inport  Port=3  DataType=double  OutDataType=sfix(16)  OutScaling=2^0  OutDataTypeStr=double
  Rx_Data : Inport  Port=4  DataType=double  OutDataType=sfix(16)  OutScaling=2^0  OutDataTypeStr=double
  Tx_ID : Inport  Port=5  DataType=double  OutDataType=sfix(16)  OutScaling=2^0  OutDataTypeStr=double
  Tx_RTR : Inport  Port=6  DataType=double  OutDataType=sfix(16)  OutScaling=2^0  OutDataTypeStr=double
  Tx_Data : Inport  Port=7  DataType=double  OutDataType=sfix(16)  OutScaling=2^0  OutDataTypeStr=double
  AAA___ : Subsystem  LoadFcn=des_subsystemsupportblock(gcb, 'load');  InitFcn=des_subsystemsupportblock(gcb, 'init');  StartFcn=des_subsystemsupportblock(gcb, 'start');  StopFcn=des_subsystemsupportblock(gcb, 'stop');
      settings: CopyFcn=des_subsystemsupportblock(gcb, 'copy');  DeleteFcn=des_subsystemsupportblock(gcb, 'delete');  UndoDeleteFcn=des_subsystemsupportblock(gcb, 'undodelete');  ModelCloseFcn=des_subsystemsupportblock(gcb, 'modelclose');  PreSaveFcn=des_subsystemsupportblock(gcb, 'presave');  NameChangeFcn=des_subsystemsupportblock(gcb, 'namechange');  OpenFcn=des_subsystemsupportblock(gcb, 'open');  ParentCloseFcn=des_subsystemsupportblock(gcb, 'parentclose');
  Mux : Mux  Inputs=8
  __fcn_ss__ : Subsystem  TreatAsAtomicUnit=on
      settings: PropExecContextOutsideSubsystem=on
  c_Loss : Constant  Value=0  OutDataType=sfix(16)  OutScaling=2^0
  c_Rx_Data : Constant  OutDataType=sfix(16)  OutScaling=2^0
  c_Rx_ID : Constant  Value=0  OutDataType=sfix(16)  OutScaling=2^0
  c_Rx_RTR : Constant  Value=0  OutDataType=sfix(16)  OutScaling=2^0
  c_Tx_Data : Constant  Value=0  OutDataType=sfix(16)  OutScaling=2^0
  c_Tx_ID : Constant  Value=0  OutDataType=sfix(16)  OutScaling=2^0
  c_Tx_RTR : Constant  Value=0  OutDataType=sfix(16)  OutScaling=2^0
  f_Loss : simeventstranslate1/Signal-Based Event to Function-Call Event  Priority=1  SystemSampleTime=-1  GenerateFunctionCallUpon=Sample time hit from port ts  SignalEdgeOption=Rising  EnableE1Port=on  EnableF2Port=off  EnableE2Port=off  SpecifyEventPriority=off  PriorityFunctionCall=20  FunctionCallDelayFrom=Dialog  DelayFunctionCall=0  StatNumberF1Calls=Off  StatNumberF2Calls=Off  MaskBlockType=DESS_DATA_PORT
  f_Rx_Data : simeventstranslate1/Signal-Based Event to Function-Call Event  Priority=1  SystemSampleTime=-1  GenerateFunctionCallUpon=Sample time hit from port ts  SignalEdgeOption=Rising  EnableE1Port=on  EnableF2Port=off  EnableE2Port=off  SpecifyEventPriority=off  PriorityFunctionCall=20  FunctionCallDelayFrom=Dialog  DelayFunctionCall=0  StatNumberF1Calls=Off  StatNumberF2Calls=Off  MaskBlockType=DESS_EVENT_PORT
  f_Rx_ID : simeventstranslate1/Signal-Based Event to Function-Call Event  Priority=1  SystemSampleTime=-1  GenerateFunctionCallUpon=Sample time hit from port ts  SignalEdgeOption=Rising  EnableE1Port=on  EnableF2Port=off  EnableE2Port=off  SpecifyEventPriority=off  PriorityFunctionCall=20  FunctionCallDelayFrom=Dialog  DelayFunctionCall=0  StatNumberF1Calls=Off  StatNumberF2Calls=Off  MaskBlockType=DESS_DATA_PORT
  f_Rx_RTR : simeventstranslate1/Signal-Based Event to Function-Call Event  Priority=1  SystemSampleTime=-1  GenerateFunctionCallUpon=Sample time hit from port ts  SignalEdgeOption=Rising  EnableE1Port=on  EnableF2Port=off  EnableE2Port=off  SpecifyEventPriority=off  PriorityFunctionCall=20  FunctionCallDelayFrom=Dialog  DelayFunctionCall=0  StatNumberF1Calls=Off  StatNumberF2Calls=Off  MaskBlockType=DESS_DATA_PORT
  f_Tx_Data : simeventstranslate1/Signal-Based Event to Function-Call Event  Priority=1  SystemSampleTime=-1  GenerateFunctionCallUpon=Sample time hit from port ts  SignalEdgeOption=Rising  EnableE1Port=on  EnableF2Port=off  EnableE2Port=off  SpecifyEventPriority=off  PriorityFunctionCall=200  FunctionCallDelayFrom=Dialog  DelayFunctionCall=0  StatNumberF1Calls=Off  StatNumberF2Calls=Off  MaskBlockType=DESS_DATA_PORT
  f_Tx_ID : simeventstranslate1/Signal-Based Event to Function-Call Event  Priority=1  SystemSampleTime=-1  GenerateFunctionCallUpon=Sample time hit from port ts  SignalEdgeOption=Rising  EnableE1Port=on  EnableF2Port=off  EnableE2Port=off  SpecifyEventPriority=off  PriorityFunctionCall=200  FunctionCallDelayFrom=Dialog  DelayFunctionCall=0  StatNumberF1Calls=Off  StatNumberF2Calls=Off  MaskBlockType=DESS_DATA_PORT
  f_Tx_RTR : simeventstranslate1/Signal-Based Event to Function-Call Event  Priority=1  SystemSampleTime=-1  GenerateFunctionCallUpon=Sample time hit from port ts  SignalEdgeOption=Rising  EnableE1Port=on  EnableF2Port=off  EnableE2Port=off  SpecifyEventPriority=off  PriorityFunctionCall=200  FunctionCallDelayFrom=Dialog  DelayFunctionCall=0  StatNumberF1Calls=Off  StatNumberF2Calls=Off  MaskBlockType=DESS_DATA_PORT
  ground : Ground
  Idx : Outport  OutDataType=sfix(16)  OutScaling=2^0
  ACK : Outport  Port=2  OutDataType=sfix(16)  OutScaling=2^0
  wires:
  Mux/1 -> __fcn_ss__/Trigger
  c_Rx_ID/1 -> f_Rx_ID/2
  f_Rx_ID/1 -> Mux/1
  __fcn_ss__/1(Idx) -> Idx/1
  f_Loss/1 -> Mux/2
  c_Loss/1 -> f_Loss/2
  Loss/1 -> f_Loss/1, __fcn_ss__/2(Loss)
  f_Rx_RTR/1 -> Mux/3
  c_Rx_RTR/1 -> f_Rx_RTR/2
  Rx_RTR/1 -> f_Rx_RTR/1, __fcn_ss__/3(Rx_RTR)
  f_Rx_Data/1 -> Mux/4
  c_Rx_Data/1 -> f_Rx_Data/2
  Tx_ID/1 -> f_Tx_ID/1, __fcn_ss__/5(Tx_ID)
  f_Tx_ID/1 -> Mux/5
  c_Tx_ID/1 -> f_Tx_ID/2
  Tx_RTR/1 -> f_Tx_RTR/1, __fcn_ss__/6(Tx_RTR)
  f_Tx_RTR/1 -> Mux/6
  c_Tx_RTR/1 -> f_Tx_RTR/2
  Tx_Data/1 -> f_Tx_Data/1, __fcn_ss__/7(Tx_Data)
  f_Tx_Data/1 -> Mux/7
  c_Tx_Data/1 -> f_Tx_Data/2
  __fcn_ss__/2(ACK) -> ACK/1
  Rx_ID/1 -> f_Rx_ID/1, __fcn_ss__/1(Rx_ID)
  ground/1 -> Mux/8
  Rx_Data/1 -> f_Rx_Data/1, __fcn_ss__/4(Rx_Data)

== system sedemo_absbrake_can/CANbus/Background Traffic/Flow Controller ==
  note: PLEASE DO NOT MODIFY ANYTHING IN THIS SUBSYSTEM.
      | This Subsystem is automatically generated and
      | managed by the Discrete Event Subsystem.
  busy : Inport  DataType=double  OutDataType=sfix(16)  OutScaling=2^0  OutDataTypeStr=double
  AAA___ : Subsystem  LoadFcn=des_subsystemsupportblock(gcb, 'load');  InitFcn=des_subsystemsupportblock(gcb, 'init');  StartFcn=des_subsystemsupportblock(gcb, 'start');  StopFcn=des_subsystemsupportblock(gcb, 'stop');
      settings: CopyFcn=des_subsystemsupportblock(gcb, 'copy');  DeleteFcn=des_subsystemsupportblock(gcb, 'delete');  UndoDeleteFcn=des_subsystemsupportblock(gcb, 'undodelete');  ModelCloseFcn=des_subsystemsupportblock(gcb, 'modelclose');  PreSaveFcn=des_subsystemsupportblock(gcb, 'presave');  NameChangeFcn=des_subsystemsupportblock(gcb, 'namechange');  OpenFcn=des_subsystemsupportblock(gcb, 'open');  ParentCloseFcn=des_subsystemsupportblock(gcb, 'parentclose');
  Mux : Mux  Inputs=1
  __fcn_ss__ : Subsystem  TreatAsAtomicUnit=on
      settings: PropExecContextOutsideSubsystem=on
  c_busy : Constant  OutDataType=sfix(16)  OutScaling=2^0
  f_busy : simeventstranslate1/Signal-Based Event to Function-Call Event  Priority=1  SystemSampleTime=-1  GenerateFunctionCallUpon=Sample time hit from port ts  SignalEdgeOption=Rising  EnableE1Port=on  EnableF2Port=off  EnableE2Port=off  SpecifyEventPriority=on  PriorityFunctionCall=2100  FunctionCallDelayFrom=Dialog  DelayFunctionCall=0  StatNumberF1Calls=Off  StatNumberF2Calls=Off  MaskBlockType=DESS_EVENT_PORT
  en : Outport  OutDataType=sfix(16)  OutScaling=2^0
  wires:
  Mux/1 -> __fcn_ss__/Trigger
  c_busy/1 -> f_busy/2
  f_busy/1 -> Mux/1
  __fcn_ss__/1(en) -> en/1
  busy/1 -> f_busy/1, __fcn_ss__/1(busy)

== system sedemo_absbrake_can/CANbus/Background Traffic/background1 ==

== system sedemo_absbrake_can/CANbus/Background Traffic/background2 ==

== system sedemo_absbrake_can/CANbus/Background Traffic/background3 ==

== system sedemo_absbrake_can/CANbus/Background Traffic/background4 ==

== system sedemo_absbrake_can/CANbus/CAN BUS Arbitration/Flow Controller ==
  note: PLEASE DO NOT MODIFY ANYTHING IN THIS SUBSYSTEM.
      | This Subsystem is automatically generated and
      | managed by the Discrete Event Subsystem.
  Busy : Inport  DataType=double  OutDataType=sfix(16)  OutScaling=2^0  OutDataTypeStr=double
  AAA___ : Subsystem  LoadFcn=des_subsystemsupportblock(gcb, 'load');  InitFcn=des_subsystemsupportblock(gcb, 'init');  StartFcn=des_subsystemsupportblock(gcb, 'start');  StopFcn=des_subsystemsupportblock(gcb, 'stop');
      settings: CopyFcn=des_subsystemsupportblock(gcb, 'copy');  DeleteFcn=des_subsystemsupportblock(gcb, 'delete');  UndoDeleteFcn=des_subsystemsupportblock(gcb, 'undodelete');  ModelCloseFcn=des_subsystemsupportblock(gcb, 'modelclose');  PreSaveFcn=des_subsystemsupportblock(gcb, 'presave');  NameChangeFcn=des_subsystemsupportblock(gcb, 'namechange');  OpenFcn=des_subsystemsupportblock(gcb, 'open');  ParentCloseFcn=des_subsystemsupportblock(gcb, 'parentclose');
  Mux : Mux  Inputs=3
  __fcn_ss__ : Subsystem  TreatAsAtomicUnit=on
      settings: PropExecContextOutsideSubsystem=on
  c_Busy : Constant  OutDataType=sfix(16)  OutScaling=2^0
  f_Busy : simeventstranslate1/Signal-Based Event to Function-Call Event  Priority=1  SystemSampleTime=-1  GenerateFunctionCallUpon=Sample time hit from port ts  SignalEdgeOption=Rising  EnableE1Port=on  EnableF2Port=off  EnableE2Port=off  SpecifyEventPriority=on  PriorityFunctionCall=2200  FunctionCallDelayFrom=Dialog  DelayFunctionCall=0  StatNumberF1Calls=Off  StatNumberF2Calls=Off  MaskBlockType=DESS_EVENT_PORT
  ground : Ground
  ground1 : Ground
  open : Outport  OutDataType=sfix(16)  OutScaling=2^0
  wires:
  ground1/1 -> Mux/3
  ground/1 -> Mux/2
  __fcn_ss__/1(open) -> open/1
  f_Busy/1 -> Mux/1
  c_Busy/1 -> f_Busy/2
  Mux/1 -> __fcn_ss__/Trigger
  Busy/1 -> f_Busy/1, __fcn_ss__/1(Busy)

== system sedemo_absbrake_can/CANbus/CAN BUS Arbitration/background4 ==

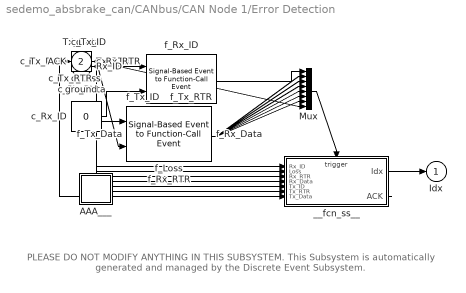
== system sedemo_absbrake_can/CANbus/CAN Node 1/Error Detection ==
  note: PLEASE DO NOT MODIFY ANYTHING IN THIS SUBSYSTEM.
      | This Subsystem is automatically generated and
      | managed by the Discrete Event Subsystem.
  Rx_ID : Inport  DataType=double  OutDataType=sfix(16)  OutScaling=2^0  OutDataTypeStr=double
  Loss : Inport  Port=2  DataType=double  OutDataType=sfix(16)  OutScaling=2^0  OutDataTypeStr=double
  Rx_RTR : Inport  Port=3  DataType=double  OutDataType=sfix(16)  OutScaling=2^0  OutDataTypeStr=double
  Rx_Data : Inport  Port=4  DataType=double  OutDataType=sfix(16)  OutScaling=2^0  OutDataTypeStr=double
  Tx_ID : Inport  Port=5  DataType=double  OutDataType=sfix(16)  OutScaling=2^0  OutDataTypeStr=double
  Tx_RTR : Inport  Port=6  DataType=double  OutDataType=sfix(16)  OutScaling=2^0  OutDataTypeStr=double
  Tx_Data : Inport  Port=7  DataType=double  OutDataType=sfix(16)  OutScaling=2^0  OutDataTypeStr=double
  AAA___ : Subsystem  LoadFcn=des_subsystemsupportblock(gcb, 'load');  InitFcn=des_subsystemsupportblock(gcb, 'init');  StartFcn=des_subsystemsupportblock(gcb, 'start');  StopFcn=des_subsystemsupportblock(gcb, 'stop');
      settings: CopyFcn=des_subsystemsupportblock(gcb, 'copy');  DeleteFcn=des_subsystemsupportblock(gcb, 'delete');  UndoDeleteFcn=des_subsystemsupportblock(gcb, 'undodelete');  ModelCloseFcn=des_subsystemsupportblock(gcb, 'modelclose');  PreSaveFcn=des_subsystemsupportblock(gcb, 'presave');  NameChangeFcn=des_subsystemsupportblock(gcb, 'namechange');  OpenFcn=des_subsystemsupportblock(gcb, 'open');  ParentCloseFcn=des_subsystemsupportblock(gcb, 'parentclose');
  Mux : Mux  Inputs=8
  __fcn_ss__ : Subsystem  TreatAsAtomicUnit=on
      settings: PropExecContextOutsideSubsystem=on
  c_Loss : Constant  Value=0  OutDataType=sfix(16)  OutScaling=2^0
  c_Rx_Data : Constant  OutDataType=sfix(16)  OutScaling=2^0
  c_Rx_ID : Constant  Value=0  OutDataType=sfix(16)  OutScaling=2^0
  c_Rx_RTR : Constant  Value=0  OutDataType=sfix(16)  OutScaling=2^0
  c_Tx_Data : Constant  Value=0  OutDataType=sfix(16)  OutScaling=2^0
  c_Tx_ID : Constant  Value=0  OutDataType=sfix(16)  OutScaling=2^0
  c_Tx_RTR : Constant  Value=0  OutDataType=sfix(16)  OutScaling=2^0
  f_Loss : simeventstranslate1/Signal-Based Event to Function-Call Event  Priority=1  SystemSampleTime=-1  GenerateFunctionCallUpon=Sample time hit from port ts  SignalEdgeOption=Rising  EnableE1Port=on  EnableF2Port=off  EnableE2Port=off  SpecifyEventPriority=off  PriorityFunctionCall=20  FunctionCallDelayFrom=Dialog  DelayFunctionCall=0  StatNumberF1Calls=Off  StatNumberF2Calls=Off  MaskBlockType=DESS_DATA_PORT
  f_Rx_Data : simeventstranslate1/Signal-Based Event to Function-Call Event  Priority=1  SystemSampleTime=-1  GenerateFunctionCallUpon=Sample time hit from port ts  SignalEdgeOption=Rising  EnableE1Port=on  EnableF2Port=off  EnableE2Port=off  SpecifyEventPriority=off  PriorityFunctionCall=20  FunctionCallDelayFrom=Dialog  DelayFunctionCall=0  StatNumberF1Calls=Off  StatNumberF2Calls=Off  MaskBlockType=DESS_EVENT_PORT
  f_Rx_ID : simeventstranslate1/Signal-Based Event to Function-Call Event  Priority=1  SystemSampleTime=-1  GenerateFunctionCallUpon=Sample time hit from port ts  SignalEdgeOption=Rising  EnableE1Port=on  EnableF2Port=off  EnableE2Port=off  SpecifyEventPriority=off  PriorityFunctionCall=20  FunctionCallDelayFrom=Dialog  DelayFunctionCall=0  StatNumberF1Calls=Off  StatNumberF2Calls=Off  MaskBlockType=DESS_DATA_PORT
  f_Rx_RTR : simeventstranslate1/Signal-Based Event to Function-Call Event  Priority=1  SystemSampleTime=-1  GenerateFunctionCallUpon=Sample time hit from port ts  SignalEdgeOption=Rising  EnableE1Port=on  EnableF2Port=off  EnableE2Port=off  SpecifyEventPriority=off  PriorityFunctionCall=20  FunctionCallDelayFrom=Dialog  DelayFunctionCall=0  StatNumberF1Calls=Off  StatNumberF2Calls=Off  MaskBlockType=DESS_DATA_PORT
  f_Tx_Data : simeventstranslate1/Signal-Based Event to Function-Call Event  Priority=1  SystemSampleTime=-1  GenerateFunctionCallUpon=Sample time hit from port ts  SignalEdgeOption=Rising  EnableE1Port=on  EnableF2Port=off  EnableE2Port=off  SpecifyEventPriority=off  PriorityFunctionCall=200  FunctionCallDelayFrom=Dialog  DelayFunctionCall=0  StatNumberF1Calls=Off  StatNumberF2Calls=Off  MaskBlockType=DESS_DATA_PORT
  f_Tx_ID : simeventstranslate1/Signal-Based Event to Function-Call Event  Priority=1  SystemSampleTime=-1  GenerateFunctionCallUpon=Sample time hit from port ts  SignalEdgeOption=Rising  EnableE1Port=on  EnableF2Port=off  EnableE2Port=off  SpecifyEventPriority=off  PriorityFunctionCall=200  FunctionCallDelayFrom=Dialog  DelayFunctionCall=0  StatNumberF1Calls=Off  StatNumberF2Calls=Off  MaskBlockType=DESS_DATA_PORT
  f_Tx_RTR : simeventstranslate1/Signal-Based Event to Function-Call Event  Priority=1  SystemSampleTime=-1  GenerateFunctionCallUpon=Sample time hit from port ts  SignalEdgeOption=Rising  EnableE1Port=on  EnableF2Port=off  EnableE2Port=off  SpecifyEventPriority=off  PriorityFunctionCall=200  FunctionCallDelayFrom=Dialog  DelayFunctionCall=0  StatNumberF1Calls=Off  StatNumberF2Calls=Off  MaskBlockType=DESS_DATA_PORT
  ground : Ground
  Idx : Outport  OutDataType=sfix(16)  OutScaling=2^0
  ACK : Outport  Port=2  OutDataType=sfix(16)  OutScaling=2^0
  wires:
  ground/1 -> Mux/8
  Rx_ID/1 -> __fcn_ss__/1(Rx_ID), f_Rx_ID/1
  __fcn_ss__/2(ACK) -> ACK/1
  c_Tx_Data/1 -> f_Tx_Data/2
  f_Tx_Data/1 -> Mux/7
  Tx_Data/1 -> __fcn_ss__/7(Tx_Data), f_Tx_Data/1
  c_Tx_RTR/1 -> f_Tx_RTR/2
  f_Tx_RTR/1 -> Mux/6
  Tx_RTR/1 -> __fcn_ss__/6(Tx_RTR), f_Tx_RTR/1
  c_Tx_ID/1 -> f_Tx_ID/2
  f_Tx_ID/1 -> Mux/5
  Tx_ID/1 -> __fcn_ss__/5(Tx_ID), f_Tx_ID/1
  c_Rx_Data/1 -> f_Rx_Data/2
  f_Rx_Data/1 -> Mux/4
  Rx_RTR/1 -> __fcn_ss__/3(Rx_RTR), f_Rx_RTR/1
  c_Rx_RTR/1 -> f_Rx_RTR/2
  f_Rx_RTR/1 -> Mux/3
  Loss/1 -> __fcn_ss__/2(Loss), f_Loss/1
  c_Loss/1 -> f_Loss/2
  f_Loss/1 -> Mux/2
  __fcn_ss__/1(Idx) -> Idx/1
  f_Rx_ID/1 -> Mux/1
  c_Rx_ID/1 -> f_Rx_ID/2
  Mux/1 -> __fcn_ss__/Trigger
  Rx_Data/1 -> f_Rx_Data/1, __fcn_ss__/4(Rx_Data)
